simulink model "ex_modeling_component_reuse"  (Simulink 10.0)
settings: Solver=VariableStepAuto  StartTime=0.0  StopTime=30  RelTol=1e-3
PreLoadFcn:
  | run(fullfile(matlabroot,'examples','simulink','main',...
  | 'ex_modeling_data_mechanical_system.m'))
  | 
  | run(fullfile(matlabroot,'examples','simulink','main',...
  | 'ex_modeling_bus_objects.m'))
libraries: ex_modeling_library x2
settings Model: Creator=The MathWorks, Inc.  LastModifiedBy=bhisma
settings DataIOCC: SaveFormat=Dataset
settings OptimizationCC: LifeSpan=auto
settings DebuggingCC: UnderspecifiedInitializationDetection=Simplified  MergeDetectMultiDrivingBlocksExec=error  ModelReferenceExtraNoncontSigs=warning  PregeneratedLibrarySubsystemCodeDiagnostic=none  SFUnexpectedBacktrackingDiag=error  SFNoUnconditionalDefaultTransitionDiag=error  SFExecutionAtInitializationDiag=warning
settings HardwareCC: ProdBitPerPointer=64  ProdBitPerSizeT=64  ProdBitPerPtrDiffT=64  ProdLargestAtomicFloat=Float  ProdIntDivRoundTo=Zero  ProdEndianess=LittleEndian  ProdWordSize=64  ProdHWDeviceType=Intel->x86-64 (Windows64)
settings ModelReferenceCC: PropagateSignalLabelsOutOfModel=on
settings CodeAppCC: StateflowObjectComments=off
settings GRTTargetCC: TargetLangStandard=C99 (ISO)  CombineOutputUpdateFcns=on  GRTInterface=off
settings ConfigComp: CovMetricSettings=dwe  CovHtmlReporting=off  CovSaveCumulativeToWorkspaceVar=off  CovSaveSingleToWorkspaceVar=off

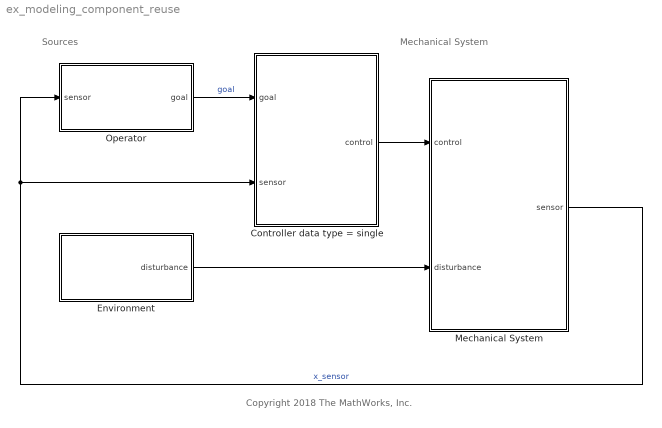
== system ex_modeling_component_reuse ==
  note: Mechanical System
  note: Sources
  note: Copyright 2018 The MathWorks, Inc.
  Controller data type = single : Subsystem
  Environment : Subsystem
  Mechanical System : Subsystem
  Operator : Subsystem
  wires:
  Mechanical System/1(sensor) -> Controller data type = single/2(sensor), Operator/1(sensor)  "x_sensor"
  Environment/1(disturbance) -> Mechanical System/2(disturbance)
  Operator/1(goal) -> Controller data type = single/1(goal)  "goal"
  Controller data type = single/1(control) -> Mechanical System/1(control)

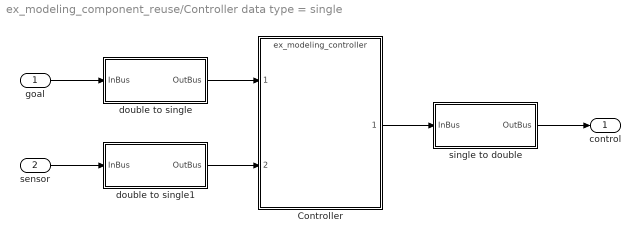
== system ex_modeling_component_reuse/Controller data type = single ==
  goal : Inport
  sensor : Inport  Port=2
  Controller : ModelReference  ModelNameDialog=ex_modeling_controller  SimulationMode=Normal  ModelReferenceVersion=1.73
  double to single : Subsystem
  double to single1 : Subsystem
  single to double : Subsystem
  control : Outport  VectorParamsAs1DForOutWhenUnconnected=off
  wires:
  goal/1 -> double to single/1(InBus)
  sensor/1 -> double to single1/1(InBus)
  Controller/1 -> single to double/1(InBus)
  double to single/1(OutBus) -> Controller/1
  double to single1/1(OutBus) -> Controller/2
  single to double/1(OutBus) -> control/1

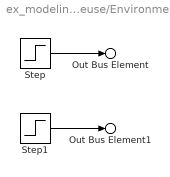
== system ex_modeling_component_reuse/Environment ==
  Step : Step  Time=10  After=10  SampleTime=0
  Step1 : Step  Time=20  After=10  SampleTime=0
  Out Bus Element : Outport  VectorParamsAs1DForOutWhenUnconnected=off  PortName=disturbance  Element=F1
  Out Bus Element1 : Outport  VectorParamsAs1DForOutWhenUnconnected=off  PortName=disturbance  Element=F2
  wires:
  Step/1 -> Out Bus Element/1
  Step1/1 -> Out Bus Element1/1

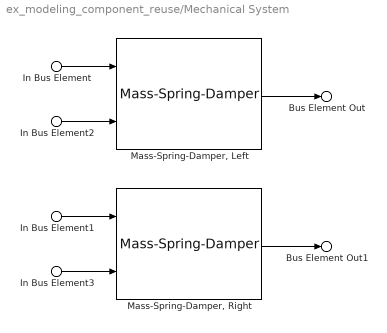
== system ex_modeling_component_reuse/Mechanical System ==
  In Bus Element : Inport  PortName=control  Element=F1
  In Bus Element1 : Inport  PortName=control  Element=F2
  In Bus Element2 : Inport  Port=2  PortName=disturbance  Element=F1
  In Bus Element3 : Inport  Port=2  PortName=disturbance  Element=F2
  "Mass-Spring-Damper, Left" : ex_modeling_library/Mass-Spring-Damper  SystemSampleTime=-1
  "Mass-Spring-Damper, Right" : ex_modeling_library/Mass-Spring-Damper  SystemSampleTime=-1
  Bus Element Out : Outport  VectorParamsAs1DForOutWhenUnconnected=off  PortName=sensor  Element=x1
  Bus Element Out1 : Outport  VectorParamsAs1DForOutWhenUnconnected=off  PortName=sensor  Element=x2
  wires:
  In Bus Element/1 -> "Mass-Spring-Damper, Left"/1
  In Bus Element1/1 -> "Mass-Spring-Damper, Right"/1
  In Bus Element2/1 -> "Mass-Spring-Damper, Left"/2
  In Bus Element3/1 -> "Mass-Spring-Damper, Right"/2
  "Mass-Spring-Damper, Left"/1 -> Bus Element Out/1
  "Mass-Spring-Damper, Right"/1 -> Bus Element Out1/1

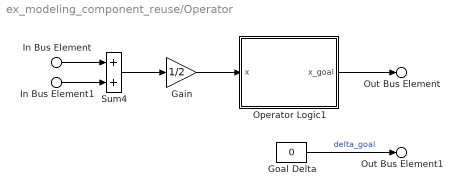
== system ex_modeling_component_reuse/Operator ==
  In Bus Element1 : Inport  PortName=sensor  Element=x2
  In Bus Element : Inport  PortName=sensor  Element=x1
  Gain : Gain  Gain=1/2
  Goal Delta : Constant  Value=0
  Operator Logic1 : Stateflow chart  TreatAsAtomicUnit=on
  Sum4 : Sum
  Out Bus Element : Outport  VectorParamsAs1DForOutWhenUnconnected=off  PortName=goal  Element=x_goal
  Out Bus Element1 : Outport  VectorParamsAs1DForOutWhenUnconnected=off  PortName=goal  Element=delta_goal
  wires:
  Gain/1 -> Operator Logic1/1(x)
  Operator Logic1/1(x_goal) -> Out Bus Element/1
  Goal Delta/1 -> Out Bus Element1/1  "delta_goal"
  In Bus Element1/1 -> Sum4/2
  In Bus Element/1 -> Sum4/1
  Sum4/1 -> Gain/1

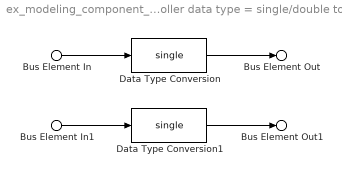
== system ex_modeling_component_reuse/Controller data type = single/double to single ==
  Bus Element In1 : Inport  PortName=InBus  Element=delta_goal
  Bus Element In : Inport  PortName=InBus  Element=x_goal
  Data Type Conversion : DataTypeConversion  OutDataTypeStr=single
  Data Type Conversion1 : DataTypeConversion  OutDataTypeStr=single
  Bus Element Out : Outport  VectorParamsAs1DForOutWhenUnconnected=off  PortName=OutBus  Element=x_goal
  Bus Element Out1 : Outport  VectorParamsAs1DForOutWhenUnconnected=off  PortName=OutBus  Element=delta_goal
  wires:
  Bus Element In/1 -> Data Type Conversion/1
  Data Type Conversion/1 -> Bus Element Out/1
  Data Type Conversion1/1 -> Bus Element Out1/1
  Bus Element In1/1 -> Data Type Conversion1/1

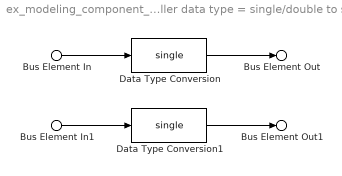
== system ex_modeling_component_reuse/Controller data type = single/double to single1 ==
  Bus Element In1 : Inport  PortName=InBus  Element=x2
  Bus Element In : Inport  PortName=InBus  Element=x1
  Data Type Conversion : DataTypeConversion  OutDataTypeStr=single
  Data Type Conversion1 : DataTypeConversion  OutDataTypeStr=single
  Bus Element Out : Outport  VectorParamsAs1DForOutWhenUnconnected=off  PortName=OutBus  Element=x1
  Bus Element Out1 : Outport  VectorParamsAs1DForOutWhenUnconnected=off  PortName=OutBus  Element=x2
  wires:
  Bus Element In1/1 -> Data Type Conversion1/1
  Data Type Conversion1/1 -> Bus Element Out1/1
  Data Type Conversion/1 -> Bus Element Out/1
  Bus Element In/1 -> Data Type Conversion/1

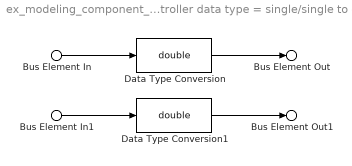
== system ex_modeling_component_reuse/Controller data type = single/single to double ==
  Bus Element In : Inport  PortName=InBus  Element=F1
  Bus Element In1 : Inport  PortName=InBus  Element=F2
  Data Type Conversion : DataTypeConversion  OutDataTypeStr=double
  Data Type Conversion1 : DataTypeConversion  OutDataTypeStr=double
  Bus Element Out : Outport  VectorParamsAs1DForOutWhenUnconnected=off  PortName=OutBus  Element=F1
  Bus Element Out1 : Outport  VectorParamsAs1DForOutWhenUnconnected=off  PortName=OutBus  Element=F2
  wires:
  Bus Element In/1 -> Data Type Conversion/1
  Data Type Conversion/1 -> Bus Element Out/1
  Data Type Conversion1/1 -> Bus Element Out1/1
  Bus Element In1/1 -> Data Type Conversion1/1

== stateflow chart Operator/Operator Logic1 ==
  state wait
    entry: x_goal = 0;
  state FirstOperation
    entry: x_goal = 2;
  state SecondOperation
    entry: x_goal = 1;
  wait -> FirstOperation : after(2,sec)
  FirstOperation -> SecondOperation : [x>2]
  (default) -> wait
  data: x input double; x_goal output double
